simulink model "Exercitiul_3_simulink"  (R2021b)
settings: Solver=VariableStepAuto  StartTime=0.0  StopTime=10.0  RelTol=1e-3

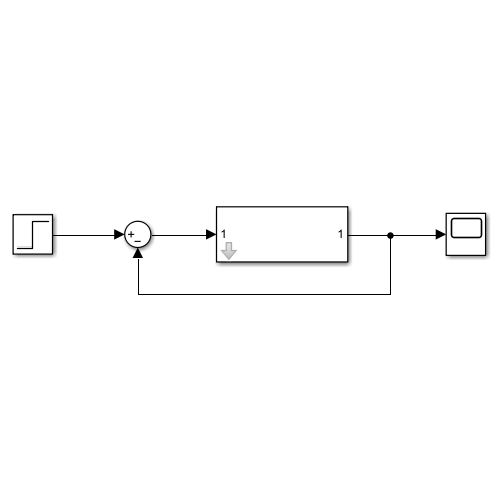
[thumbnail: Simulink's stored preview of the top-level diagram]
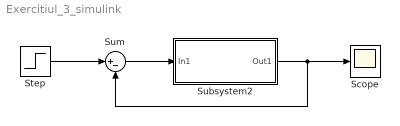
== system Exercitiul_3_simulink ==
  Scope : Scope
  Step : Step  SampleTime=0
  Subsystem2 : Subsystem  mask{a=12.25}
      mask prompts: a "a="
      mask init:
      | if str2num(get_param(gcb, 'a'))<8 || str2num(get_param(gcb, 'a'))<8str2num(get_param(gcb, 'a'))>4
      | error('a nu se afla in intervalul [6,8]')
      | end
      mask Callback a:
      | if str2num(get_param(gcb,'a'))<0
      |     error('Valoare negativa')
      | end
  Sum : Sum  Inputs=|+-
  wires:
  Subsystem2/1(Out1) -> Sum/2, Scope/1
  Step/1 -> Sum/1
  Sum/1 -> Subsystem2/1(In1)

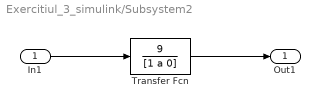
== system Exercitiul_3_simulink/Subsystem2 ==
  In1 : Inport
  Transfer Fcn : TransferFcn  Numerator=[9]  Denominator=[1 a 0]
  Out1 : Outport
  wires:
  In1/1 -> Transfer Fcn/1
  Transfer Fcn/1 -> Out1/1
